simulink model "washingmachine"  (R2024b)
settings: Solver=VariableStepAuto  StartTime=0.0  StopTime=10.0  RelTol=1e-3
settings Model: Creator=Krishna K S  LastModifiedBy=Krishna K S

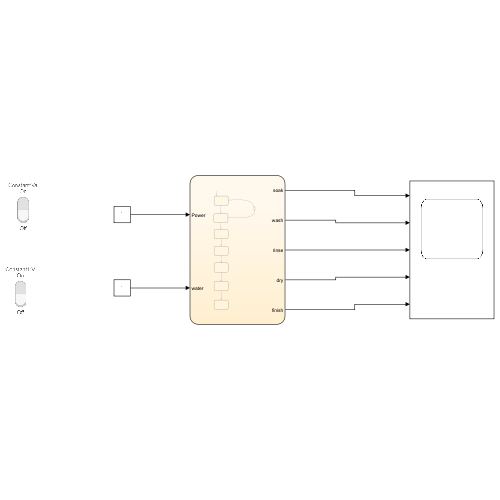
[thumbnail: Simulink's stored preview of the top-level diagram]
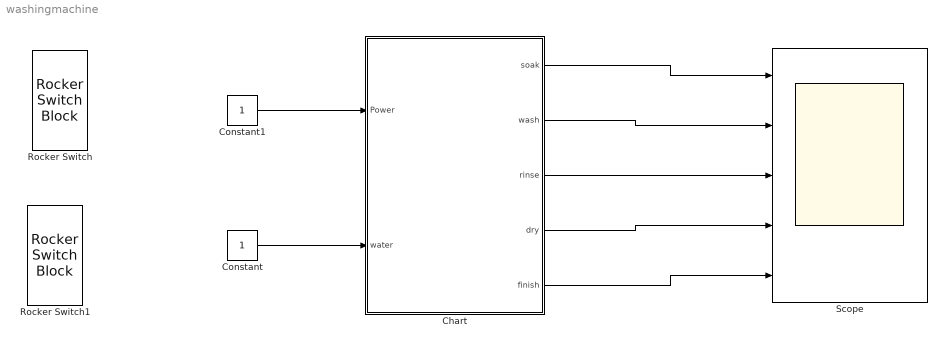
== system washingmachine ==
  Chart : Stateflow chart  TreatAsAtomicUnit=on
  Constant : Constant
  Constant1 : Constant
  Rocker Switch : RockerSwitchBlock
      settings: Values={{'Off', 'On'}, [0 1]}
  Rocker Switch1 : RockerSwitchBlock
      settings: Values={{'Off', 'On'}, [0 1]}
  Scope : Scope  NumInputPorts=5
  wires:
  Constant1/1 -> Chart/1(Power)
  Constant/1 -> Chart/2(water)
  Chart/1(soak) -> Scope/1
  Chart/2(wash) -> Scope/2
  Chart/3(rinse) -> Scope/3
  Chart/4(dry) -> Scope/4
  Chart/5(finish) -> Scope/5

== stateflow chart washingmachine/Chart ==
  state Power
  state water
  state soak
    entry:soak=1
  state wash
    entry:wash=1
  state rinse
    entry:rinse=1
  state dry
    entry:dry=1
  state finish
    entry:finish=1
  (default) -> Power
  Power -> (junction 15) [order 1] : [Power==0]
  Power -> water [order 2]
  water -> (junction 15) [order 2] : [water==0]
  water -> soak [order 1] : [water==1]
  soak -> wash : [after(200,sec)]
  wash -> rinse : [after(100,sec)]
  rinse -> dry : [after(20,sec)]
  dry -> finish : [after(50,sec)]
  data: soak output; Power input; water input; wash output; rinse output; dry output; finish output
